simulink model "parte1_eje7_Control_PF"  (R2017b)
settings: Solver=VariableStepAuto  StartTime=0.0  StopTime=120  RelTol=1e-3
values from neighbouring files (symbols this model uses):
  b = 0.0425    [parte1_eje7_Control_PF_datos.m]
  Ki = 0.09    [parte1_eje7_Control_PF_datos.m]
  Kps = 100    [parte1_eje7_Control_PF_datos.m]
  R = rlocus(G,K)    [parte1_eje11_lugarderaices.m]    (also in parte1_eje1_circuitoRC.m = 10; parte1_eje2_circuitoRLC.m = 10000; parte1_eje4_SScircuitoRLC.m = 100; parte1_eje5_ft_circuitoRLC.m = 100)
  Tps = 20    [parte1_eje7_Control_PF_datos.m]
  Tt = 0.5    [parte1_eje7_Control_PF_datos.m]
undefined symbols (not defined in the file or in its folder): Tsg
settings Model: Creator=N. Quintanilla  LastModifiedBy=cjuar
settings CodeAppCC: StateflowObjectComments=on

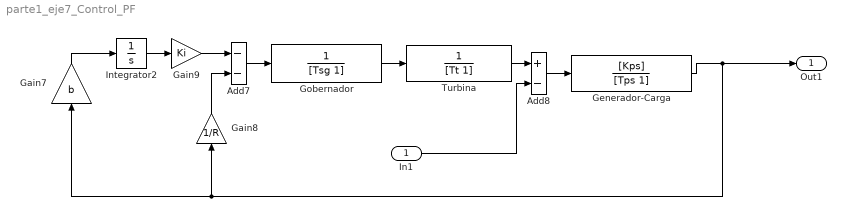
== system parte1_eje7_Control_PF ==
  In1 : Inport
  " Generador-Carga" : TransferFcn  Numerator=[Kps]  Denominator=[Tps 1]
  Add7 : Sum  Inputs=--
  Add8 : Sum  Inputs=+-
  Gain7 : Gain  Gain=b
  Gain8 : Gain  Gain=1/R
  Gain9 : Gain  Gain=Ki
  Gobernador : TransferFcn  Denominator=[Tsg 1]
  Integrator2 : Integrator
  "Turbina " : TransferFcn  Denominator=[Tt 1]
  Out1 : Outport
  wires:
  "Turbina "/1 -> Add8/1
  In1/1 -> Add8/2
  Gain9/1 -> Add7/1
  Add8/1 -> " Generador-Carga"/1
  Gain7/1 -> Integrator2/1
  Integrator2/1 -> Gain9/1
  Gain8/1 -> Add7/2
  " Generador-Carga"/1 -> Out1/1, Gain8/1, Gain7/1
  Add7/1 -> Gobernador/1
  Gobernador/1 -> "Turbina "/1
